simulink model "stabilizer_bar_repair"  (R2023a)
settings: Solver=ode4  StartTime=0  StopTime=t_final  FixedStep=Ts_plant  MaxStep=0.001  RelTol=1e-3
InitFcn:
  | run(fullfile(fileparts(get_param(bdroot,'FileName')),'a001_new_Design_LQR_Controller.m'));
values from neighbouring files (symbols this model uses):
  entry_cfg = rmfield(entry_bank_source,{'labels','source_hashes','note','source_par_sha256'})    [a001_new_Design_LQR_Controller.m]
  path_geometry = repair_build_geometry(path_cfg)    [a001_new_Design_LQR_Controller.m]
  path_Q = diag([10,10,2])    [a001_new_Design_LQR_Controller.m]
  path_R = diag([100,100,10])    [a001_new_Design_LQR_Controller.m]
  repair_cfg = struct    [a001_new_Design_LQR_Controller.m]
  repair_simfile = 'C:\Users\Public\Documents\CarSim2020.0_Data\Extensions\Simulink\00carsim_workspace\009\simfile.sim'    [a001_new_Design_LQR_Controller.m]
  Ts = 0.01    [a001_new_Design_LQR_Controller.m]
  Ts_plant = 0.0005    [a001_new_Design_LQR_Controller.m]
undefined symbols (not defined in the file or in its folder): path_cfg
(part 2 of 2)

== matlab function stabilizer_bar_repair/EntryLocalMode/EntryLocalControl ==
  settings: updateMethod=DISCRETE  sampleTime=Ts
  data: y input size=[50 1]; command output size=[5 1]; t input; diag output size=[70 1]; entry_cfg parameter; repair_cfg parameter
function [command,diag] = entry_control(y,t,entry_cfg, repair_cfg)
%#codegen
% 普通直行→滑移建立→横摆/负侧偏建立→局部维持，100Hz只更新一次状态。
% y为CarSim原50路采样输出，轮序FL/FR/RL/RR；t为仿真时间s。
% entry_cfg含实测工作点/增益、接管范围和执行预算；repair_cfg含统一车辆参数。
% command=[前轮角rad;四轮矩Nm]；后级0.5ms执行器产生一致转角与转角速度。
% 禁止在这里写车辆状态或恢复配平快照；路径LQR和式4.10不参与本支路。
persistent phase distance elapsed readyTime captureTime satTime mix mixStart mixTarget mixElapsed prepareFailed vprev wprev initialized protection
if isempty(initialized)
 phase=0;distance=0;elapsed=0;readyTime=0;captureTime=0;satTime=0;
 mix=0;mixStart=0;mixTarget=0;mixElapsed=0;prepareFailed=false;
 vprev=zeros(3,1);wprev=zeros(4,1);initialized=false;protection=false;
end
command=zeros(5,1);diag=zeros(70,1);
if repair_cfg.entry_mode==0,return;end
Ts=repair_cfg.Ts;Rw=repair_cfg.Rw;Iw=repair_cfg.Iw;
x=[hypot(y(2),y(3))/3.6;y(4)*pi/180;y(5)*pi/180; ...
 mean(y(27:28));mean(y(29:30));y(8)*pi/180;y(26)*pi/180];
omega=y(21:24)*pi/30;Fz=y(17:20);last=entry_cfg.nodes(7);
assert(all(isfinite(x))&&all(isfinite(Fz)),'Nonfinite state or normal load');
first=~initialized;
if first,vprev=entry_cfg.normal.v;wprev=omega;initialized=true;end

% 状态机：准备必须连续满足1s，接管必须连续满足0.3s；目标角/轮速历史不复位。
elapsed=elapsed+Ts;
if protection,satTime=satTime+Ts;else,satTime=0;end
inside=all(abs(x-last.x)<=entry_cfg.thresholds)&&all(Fz>0)&&satTime<.2;
if phase==0
 ready=abs(x(1)-12)<=.2&&abs(x(2))<=pi/180&&abs(x(3))<=.02;
 if ready,readyTime=readyTime+Ts;else,readyTime=0;end
 if readyTime>=1-1e-9&&~prepareFailed,phase=1;
 elseif elapsed>=10,prepareFailed=true;end
else
 if phase==1,distance=distance+max(x(1),0)*Ts;end
 if inside,captureTime=captureTime+Ts;else,captureTime=0;end
 if phase==1&&captureTime>=.3-1e-9
  phase=2;mixStart=mix;mixTarget=1;mixElapsed=0;
 end
 if (phase==2||phase==3)&&~inside&&mixTarget~=0
  phase=2;mixStart=mix;mixTarget=0;mixElapsed=0;
 end
 if phase==2
  mixElapsed=mixElapsed+Ts;mix=mixStart+(mixTarget-mixStart)*smooth5(mixElapsed/.5);
  if mixElapsed>=.5-1e-9
   if mixTarget==1,phase=3;else,phase=1;end
  end
 end
end
progress=smooth5(distance/entry_cfg.length);
if phase==0
 j=1;f=smooth5(t/2);left=entry_cfg.normal;right=entry_cfg.nodes(1);
else
 j=1;
 for k=1:6,if progress>=entry_cfg.grid(k),j=k;end,end
 f=(progress-entry_cfg.grid(j))/(entry_cfg.grid(j+1)-entry_cfg.grid(j));
 left=entry_cfg.nodes(j);right=entry_cfg.nodes(j+1);
end
refX=(1-f)*left.x+f*right.x;refV=(1-f)*left.v+f*right.v;
K=(1-f)*left.K+f*right.K;offset=(1-f)*left.offset+f*right.offset;
% 两个反馈只计算虚拟输入；在同一执行器中更新一次，不混合独立persistent轮速环。
scheduled=refV-K*(x-refX);local=last.v-last.K*(x-last.x);
request=(1-mix)*scheduled+mix*local;
refX=(1-mix)*refX+mix*last.x;refV=(1-mix)*refV+mix*last.v;
offset=(1-mix)*offset+mix*last.offset;

% 普通阶段允许滑移穿零；局部偏移和变化率均来自集中配置。
lo=[refV(1)-entry_cfg.steer_deviation;entry_cfg.slip_low];
hi=[refV(1)+entry_cfg.steer_deviation;entry_cfg.slip_high];
v=min(max(request,lo),hi);slew=[entry_cfg.steering_rate_rad_s;entry_cfg.slip_rate;entry_cfg.slip_rate];
v=min(max(v,vprev-slew*Ts),vprev+slew*Ts);vprev=v;
contact=Rw*omega./(1+y(27:30));
assert(all(isfinite(contact))&&all(contact>0),'Local wheel execution does not support reverse contact velocity');
candidate=contact/Rw.*(1+[v(2);v(2);v(3);v(3)]);
loadTorque=Rw*y(9:12)+offset;kw=entry_cfg.wheel_kw;
if first
 wd=omega;dwd=zeros(4,1);
else
 gain=kw+Iw/Ts;
 low=(-entry_cfg.torque_limit+kw*omega+Iw/Ts*wprev-loadTorque)/gain;
 high=(entry_cfg.torque_limit+kw*omega+Iw/Ts*wprev-loadTorque)/gain;
 low=max(low,wprev-entry_cfg.omega_acceleration*Ts);high=min(high,wprev+entry_cfg.omega_acceleration*Ts);
 assert(all(low<=high),'No intersection of torque and wheel acceleration budgets');
 wd=min(max(candidate,low),high);dwd=(wd-wprev)/Ts;
end
feedback=kw*(wd-omega);inertia=Iw*dwd;raw=feedback+inertia+loadTorque;
T=min(max(raw,-entry_cfg.torque_limit),entry_cfg.torque_limit);wprev=wd;
protection=any(abs(T)>=entry_cfg.torque_limit-1e-6);command=[v(1);T];
diag=[phase;progress;mix;double(inside);double(prepareFailed);readyTime;captureTime;satTime; ...
 x;refX;refV;request;v;candidate;wd;omega;feedback;inertia;loadTorque;raw;T; ...
 double(any(abs(v-request)>1e-9));double(any(abs(wd-candidate)>1e-9));double(protection);contact];
end
function h=smooth5(q)
q=min(max(q,0),1);h=10*q^3-15*q^4+6*q^5;
end

== matlab function stabilizer_bar_repair/EntryModeSelector ==
  data: newcmd input size=[5 1]; angle output; oldcmd input size=[5 1]; tfl output; tfr output; trl output; trr output; repair_cfg parameter
function [angle,tfl,tfr,trl,trr]=select_commands(newcmd,oldcmd,repair_cfg)
% 模式开关只选择执行输入；不改变两支路的数学公式。
c=oldcmd;if repair_cfg.entry_mode==1,c=newcmd;end
angle=c(1);tfl=c(2);tfr=c(3);trl=c(4);trr=c(5);
end

== matlab function stabilizer_bar_repair/EntryLocalMode/EntryForceDiagnostic ==
  settings: updateMethod=DISCRETE  sampleTime=Ts
  data: y input size=[50 1]; out output size=[20 1]; diag input size=[70 1]; repair_cfg parameter
function out=entry_force_diagnostic(y,diag,repair_cfg)
%#codegen
% 本块仅记录原三自由度逆解回代及其与实际轮胎合力的差异，不参与执行指令。
% out=[原请求4;代数回代残差3;实际轴力4;实际平面合力矩3;请求平面合力矩3;差值3]。
% 实际合力矩使用四轮Fx/Fy、前轮实测角及轮距；未包含回正力矩/外倾/三维悬架作用。
persistent history initialized
if isempty(initialized),history=zeros(4,1);initialized=false;end
out=zeros(20,1);if repair_cfg.entry_mode==0,return;end
V=diag(9);beta=diag(10);r=diag(11);ref=diag(16:18);Ts=repair_cfg.Ts;
bd=ref(2);rd=ref(3);diffs=zeros(4,1);
if initialized,diffs=([bd;beta;rd;r]-history)/Ts;end
history=[bd;beta;rd;r];initialized=true;
vdot=repair_cfg.k_V*(ref(1)-V);betadot=repair_cfg.k_beta_p*(bd-beta)+repair_cfg.k_beta_d*(diffs(1)-diffs(2));
rdot=repair_cfg.k_r_p*(rd-r)+repair_cfg.k_r_d*(diffs(3)-diffs(4));q=betadot+r;
m=repair_cfg.m;Iz=repair_cfg.Iz;a=repair_cfg.a;b=repair_cfg.b;L=a+b;
angles=[y(38:39)*pi/180;0;0];delta=mean(angles(1:2));cd=cos(delta);sd=sin(delta);
Fxf=m*vdot;Fyr=(-Iz*rdot+a*m*V*q*cos(beta)+a*m*vdot*sin(beta))/L;
Fyf=(Iz*rdot-L*Fxf*sd+b*m*V*q*cos(beta)+b*m*vdot*sin(beta))/(L*cd);
Fxr=(-L*Fxf+Iz*rdot*sd-a*m*V*q*sin(beta)*cd-b*m*V*q*sin(beta-delta)+a*m*vdot*cos(beta)*cd+b*m*vdot*cos(beta-delta))/(L*cd);
bx=Fxf*cd-Fyf*sd+Fxr;by=Fxf*sd+Fyf*cd+Fyr;mz=a*(Fxf*sd+Fyf*cd)-b*Fyr;
back=[(bx*cos(beta)+by*sin(beta))/m;(-bx*sin(beta)+by*cos(beta))/(m*V)-r;mz/Iz];
Fx=y(9:12);Fy=y(13:16);cx=Fx.*cos(angles)-Fy.*sin(angles);cy=Fx.*sin(angles)+Fy.*cos(angles);
actual=[sum(cx);sum(cy);a*sum(cy(1:2))-b*sum(cy(3:4))+repair_cfg.d/2*(cx(2)-cx(1)+cx(4)-cx(3))];
request=[bx;by;mz];out=[Fxf;Fyf;Fxr;Fyr;back-[vdot;betadot;rdot];sum(Fx(1:2));sum(Fy(1:2));sum(Fx(3:4));sum(Fy(3:4));actual;request;actual-request];
end

== matlab function stabilizer_bar_repair/MATLAB Function ==
  settings: updateMethod=DISCRETE  sampleTime=Ts
  data: Vx input; V output; Vy input
function V = cg_speed(Vx,Vy)
%#codegen
V = hypot(Vx,Vy);
end

== matlab function stabilizer_bar_repair/路径跟踪层/PoseError ==
  settings: updateMethod=DISCRETE  sampleTime=Ts
  data: X input; xi output size=[3 1]; Y input; psi input; ref input size=[14 1]
function xi = pose_error(X,Y,psi,ref)
%#codegen
% 论文式4.4~4.8：全局位置误差为实际减参考，航向误差取主值。
% 参考psi保持连续累积，只有相对误差wrap，避免参考跨圈跳变。
xi=[X-ref(1);Y-ref(2);atan2(sin(psi-ref(3)),cos(psi-ref(3)))];
end

== matlab function stabilizer_bar_repair/路径跟踪层/OnlineLQR ==
  settings: updateMethod=DISCRETE  sampleTime=Ts
  data: ref input size=[14 1]; desired output size=[3 1]; xi input size=[3 1]; diag_lqr output size=[11 1]; path_Q parameter; path_R parameter; path_cfg parameter
function [desired,diag_lqr] = path_lqr(ref,xi,path_Q,path_R,path_cfg)
% 在线LQR目标直接输出；CARE残差保留诊断，不触发自定义Assert停止。
if path_cfg.feedback_enabled==0,desired=ref(4:6);diag_lqr=zeros(11,1);return;end
coder.extrinsic('lqr');c=cos(ref(3));s=sin(ref(3));vx=ref(4);vy=ref(5);
A=[0,0,-vx*s-vy*c;0,0,vx*c-vy*s;0,0,0];B=[c,-s,0;s,c,0;0,0,1];
K=zeros(3);P=zeros(3);[K,P]=lqr(A,B,path_Q,path_R);
AP=A'*P+P*A;PB=P*B*(path_R\(B'*P));
res=norm(AP-PB+path_Q,'fro')/(1+norm(AP,'fro')+norm(PB,'fro')+norm(path_Q,'fro'));
desired=ref(4:6)-K*xi;ok=all(isfinite(K(:)))&&isfinite(res)&&res<=path_cfg.care_tol;
diag_lqr=[K(:);res;double(ok)];
end

== matlab function stabilizer_bar_repair/车辆运动控制层/StateFeasibility ==
  settings: updateMethod=DISCRETE  sampleTime=Ts
  data: actual input size=[3 1]; packet output size=[13 1]; desired input size=[3 1]; delta input; loads input size=[2 1]; blend input; path input size=[3 1]; omega input size=[4 1]; contact input size=[8 1]; accepted output size=[3 1]; diag output size=[134 1]; valid output; repair_cfg parameter
function [packet,accepted,diag,valid] = state_governor(actual,desired,delta,loads,blend,path,omega,contact,repair_cfg)
% 直接把完整LQR状态参考送入原状态控制律，不做可行候选搜索或指令缩放。
% actual=[V;beta;r]，desired=[Vx_d;Vy_d;r_d]，path=[e_y;DeltaChi;kappa]；SI单位。
% 轮胎力可达性和执行器响应交由CarSim输出反映；diag只记录直通状态。
persistent history initialized
if isempty(initialized),history=zeros(4,1);initialized=false;end
V=actual(1);beta=actual(2);r=actual(3);
Vd=hypot(desired(1),desired(2));beta_d=atan2(desired(2),desired(1));r_d=desired(3);
eV=Vd-V;eBeta=atan2(sin(beta_d-beta),cos(beta_d-beta));eR=r_d-r;
if initialized
    beta_d_dot=atan2(sin(beta_d-history(1)),cos(beta_d-history(1)))/repair_cfg.Ts;
    beta_dot=atan2(sin(beta-history(2)),cos(beta-history(2)))/repair_cfg.Ts;
    r_d_dot=(r_d-history(3))/repair_cfg.Ts;r_dot=(r-history(4))/repair_cfg.Ts;
else
    beta_d_dot=0;beta_dot=0;r_d_dot=0;r_dot=0;
end
den=1-path(3)*path(1);
beta_cmd=repair_cfg.k_beta_p*eBeta+repair_cfg.k_beta_d*(beta_d_dot-beta_dot)+ ...
    repair_cfg.k_beta*path(3)*V*cos(path(2))/den;
r_cmd=repair_cfg.k_r_p*eR+repair_cfg.k_r_d*(r_d_dot-r_dot);
V_cmd=repair_cfg.k_V*eV;
packet=[Vd;beta_d;r_d;eV;eBeta;eR;beta_cmd;r_cmd;V_cmd;beta_d_dot;beta_dot;r_d_dot;r_dot];
accepted=desired;
valid=all(isfinite([actual;desired;delta;loads;blend;path;omega;contact;packet]));
diag=nan(134,1);diag(1)=1;diag(2)=double(valid);diag(3)=1;diag(4)=NaN;diag(5)=1;
diag(6:8)=desired;diag(9:11)=accepted;diag(100)=double(~valid);diag(101)=0;
history=[beta_d;beta;r_d;r];initialized=true;
end

== matlab function stabilizer_bar_repair/车辆运动控制层/RawDynamicsInverse ==
  settings: updateMethod=DISCRETE  sampleTime=Ts
  data: packet input size=[13 1]; F output size=[4 1]; delta input; Fzr input; blend input; actual input size=[3 1]; status output; repair_cfg parameter; residual output size=[3 1]
function [F,status,residual] = inverse_block(packet,delta,Fzr,blend,actual,repair_cfg)
% 三自由度动力学逆解输出未裁剪的轴级目标力，残差仅记录、不阻止执行。
qd=packet(7)+actual(3);V=actual(1);beta=actual(2);rdot=packet(8);Vdot=packet(9);
Fxf=repair_cfg.m*Vdot;cd=cos(delta);sd=sin(delta);L=repair_cfg.a+repair_cfg.b;
Fyr=(-repair_cfg.Iz*rdot+repair_cfg.a*repair_cfg.m*V*qd*cos(beta)+ ...
    repair_cfg.a*repair_cfg.m*Vdot*sin(beta))/L;
Fyf=(repair_cfg.Iz*rdot-L*Fxf*sd+repair_cfg.b*repair_cfg.m*V*qd*cos(beta)+ ...
    repair_cfg.b*repair_cfg.m*Vdot*sin(beta))/(L*cd);
Fxr=(-L*Fxf+repair_cfg.Iz*rdot*sd-repair_cfg.a*repair_cfg.m*V*qd*sin(beta)*cd- ...
    repair_cfg.b*repair_cfg.m*V*qd*sin(beta-delta)+repair_cfg.a*repair_cfg.m*Vdot*cos(beta)*cd+ ...
    repair_cfg.b*repair_cfg.m*Vdot*cos(beta-delta))/(L*cd);
F=[Fxf;Fyf;Fxr;Fyr];bx=F(1)*cd-F(2)*sd+F(3);by=F(1)*sd+F(2)*cd+F(4);
Vdot_back=(bx*cos(beta)+by*sin(beta))/repair_cfg.m;
beta_dot_back=(-bx*sin(beta)+by*cos(beta))/(repair_cfg.m*V)-actual(3);
r_dot_back=(repair_cfg.a*(F(1)*sd+F(2)*cd)-repair_cfg.b*F(4))/repair_cfg.Iz;
residual=[Vdot_back-packet(9);beta_dot_back-packet(7);r_dot_back-packet(8)];
status=int8(0); %#ok<NASGU> 保留原状态端口，力能否实现以CarSim实际响应判断。
end

== matlab function stabilizer_bar_repair/车辆运动控制层/ForceCorrection ==
  settings: updateMethod=DISCRETE  sampleTime=Ts
  data: F input size=[4 1]; alpha output; actual input size=[3 1]; delta input; loads input size=[2 1]; wf output; wr output; Fxf output; Fxr output; diag output size=[32 1]; valid output; repair_cfg parameter
function [alpha,wf,wr,Fxf,Fxr,diag,valid] = force_block(F,actual,delta,loads,repair_cfg)
% 轴力不做摩擦圆、被动方向或前轮可达角投影；CarSim轮胎力是实际响应。
% alpha采用未饱和小侧偏斜率反算，只生成前轮指令；原始Fx用于轮速/力矩前馈。
% 轮速逆解使用载荷尺度的连续正则化，避免Fy过零时突变；它不是轮胎力/力矩限幅。
V=actual(1);beta=actual(2);r=actual(3);vx=V*cos(beta);vy=V*sin(beta);
contact=atan2(vy+repair_cfg.a*r,vx);alpha=-F(2)/repair_cfg.Caf;
vxf=vx*cos(delta)+(vy+repair_cfg.a*r)*sin(delta);
vyf=-vx*sin(delta)+(vy+repair_cfg.a*r)*cos(delta);vyr=vy-repair_cfg.b*r;
ef=repair_cfg.force_eps_frac*repair_cfg.mu*loads(1);
er=repair_cfg.force_eps_frac*repair_cfg.mu*loads(2);
wf=(vxf-vyf*F(1)*F(2)/(F(2)^2+ef^2))/repair_cfg.Rw;
wr=(vx-vyr*F(3)*F(4)/(F(4)^2+er^2))/repair_cfg.Rw;
Fxf=F(1);Fxr=F(3);valid=all(isfinite([F;actual;delta;loads;alpha;wf;wr]));
body=zeros(3,1);diag=[F;F;zeros(4,1);body;contact-alpha;contact-alpha;ef;er; ...
    ef^2/(F(2)^2+ef^2);er^2/(F(4)^2+er^2);0;0;vxf;vyf;vx;vyr;F(4)*vyr; ...
    repair_cfg.mu*loads(1);repair_cfg.mu*loads(2);NaN;double(~valid)];
end
